simulink model "hybrid_pv_wind_islanding"  (R2024b)
settings: Solver=FixedStepDiscrete  StartTime=0.0  StopTime=1.0  FixedStep=P.Ts  RelTol=1e-3
model workspace (MAT data in the model file):
  P.Sn = 20000
  P.Vll = 400
  P.fg = 50
  P.wg = 314.159265359
  P.Vdc = 800
  P.fsw = 10000
  P.Ts = 2e-06
  P.In = 28.8675134595
  P.Ipk = 40.8248290464
  P.Vpk = 326.598632371
  P.logDecim = 10
  P.Zb = 8
  P.Lb = 0.0254647908947
  P.Cb = 0.00039788735773
  P.pv.Nser = 10
  P.pv.Npar = 5
  P.pv.Vmp = 290
  P.pv.Pstc = 10657.5
  P.pv.G0 = 1000
  P.pv.G1 = 1000
  P.pv.tStep = 1000000
  P.pv.T = 25
  P.pv.Tmppt = 0.01
  P.pv.dD = 0.003
  P.pv.D0 = 0.6375
  P.pv.Dmin = 0.45
  P.pv.Dmax = 0.8
  P.wind.R = 2.7072
  P.wind.rho = 1.225
  P.wind.CpMax = 0.411
  P.wind.lamOpt = 7.954
  P.wind.v0 = 12
  P.wind.v1 = 12
  P.wind.tStep = 1000000
  P.wind.Kopt = 0.228529744693
  P.wind.wm0 = 35.2570921986
  P.wind.Prated = 10015.7207747
  P.wind.J = 10
  P.wind.pp = 4
  P.wind.Ls = 0.003
  P.wind.Imax = 90
  P.wind.KpI = 0.04
  P.wind.KiI = 12
  P.wind.D0 = 0.76
  P.lcl.ripple = 0.2
  P.lcl.L1 = 0.0016
  P.lcl.L2 = 0.0008
  P.lcl.Cf = 1.5e-05
  P.lcl.wres = 11180.3398875
  P.lcl.fres = 1779.40635854
  P.lcl.Rd = 1.98761598
  P.lcl.R1 = 0.001
  P.lcl.R2 = 0.001
  P.grid.scr = 10
  P.grid.xr = 3
  P.grid.R = 0.252982212813
  P.grid.L = 0.00241580218102
  P.pll.wn = 188.495559215
  P.pll.zeta = 0.707
  P.pll.Kp = 0.816086456932
  P.pll.Ki = 108.789726356
  P.pll.Tf = 0.00795774715459
  P.ctrl.KpI = 6
  P.ctrl.KiI = 1000
  P.ctrl.KpV = 0.5
  P.ctrl.KiV = 10
  P.ctrl.Ilim = 61.2372435696
  P.prot.uv = 0.88
  P.prot.ov = 1.1
  P.prot.uf = 49.3
  P.prot.of = 50.5
  P.prot.rocof = 2
  P.prot.Trocof = 0.001
  P.prot.tBlank = 0.3
  P.load.Qf = 1
  P.load.P = 20000
  P.load.QL = 20000
  P.load.QC = 20000
  P.tIsland = 1000000
  P.check.Cf_pct_of_Cb = 3.76991118431
  P.check.Ltot_pu = 0.0942477796077
  P.check.fres_in_range = 1
  P.check.fres_with_grid = 1257.19940734
undefined symbols (not defined in the file): DiscIntNeverNeededParam
libraries: spsSeriesRLCBranchLib x14, spsIGBTDiodeLib x8, slpidlib x5, simulink x4, spsThreePhaseBreakerLib x2, spsDiodeLib x2, spsAlphaBetaZerotodq0Lib x2, eeGeneralControl x2, spsThreePhaseVIMeasurementLib x2, spsVoltageMeasurementLib x2, spsMeanLib x1, spsabctoAlphaBetaZeroLib x1
settings Model: LastModifiedBy=subas
settings SolverCC: AlgebraicLoopSolver=LineSearch
settings DataIOCC: ReturnWorkspaceOutputs=off
settings DebuggingCC: AlgebraicLoopMsg=none  ArithmeticOperatorsInVariantConditions=warning
settings ModelReferenceCC: EnableRefExpFcnMdlSchedulingChecks=on
settings SFSimCC: SimUseLocalCustomCode=off  CustomCodeUndefinedFunction=UseInterfaceOnly
settings RTWCC: RTWUseLocalCustomCode=off  GPUComputeCapability=3.5

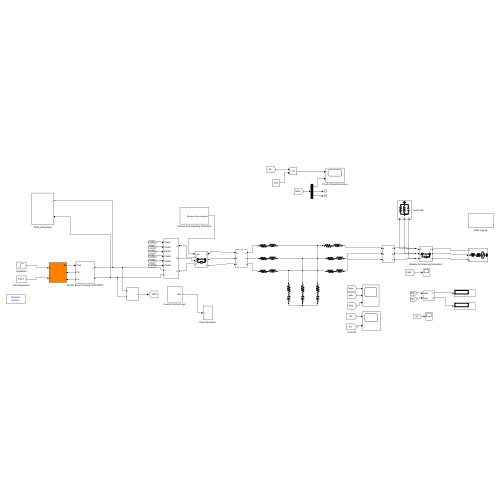
[thumbnail: Simulink's stored preview of the top-level diagram]
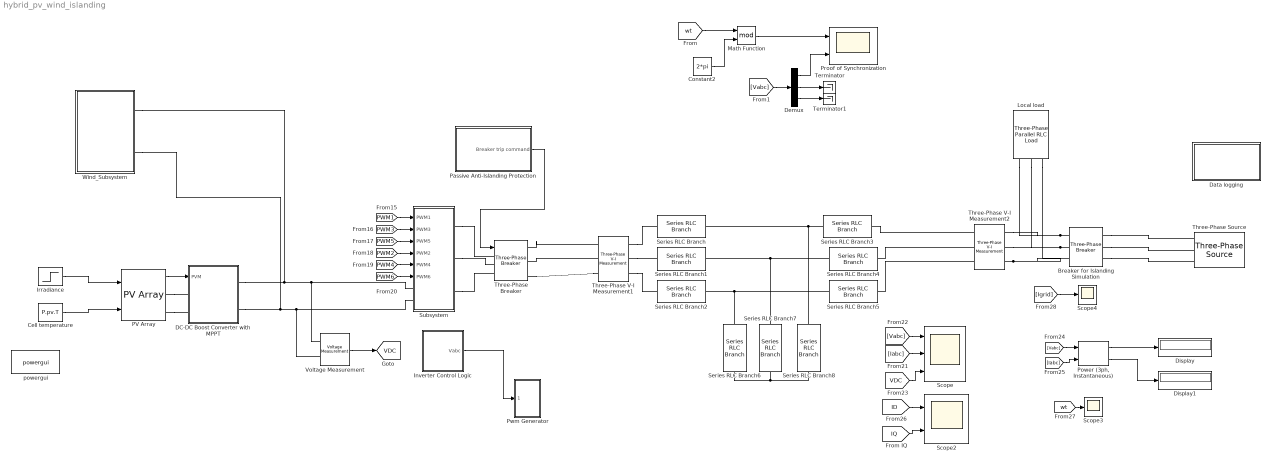
== system hybrid_pv_wind_islanding ==
  Breaker for Islanding Simulation : spsThreePhaseBreakerLib/Three-Phase Breaker  InitialState=closed  SwitchA=on  SwitchB=on  SwitchC=on  SwitchTimes=[P.tIsland]  External=off  BreakerResistance=0.01  SnubberResistance=1e6  SnubberCapacitance=inf  Measurements=None
  Cell temperature : Constant  Value=P.pv.T
  Constant2 : Constant  Value=2*pi
  DC-DC Boost Converter with MPPT : Subsystem
  Data logging : Subsystem
  Demux : Demux  Outputs=3
  Display : Display
  Display1 : Display
  Inverter Control Logic : Subsystem
  Irradiance : Step  Time=P.pv.tStep  Before=P.pv.G0  After=P.pv.G1  SampleTime=0
  Local load : spsThreePhaseParallelRLCLoadLib/Three-Phase Parallel RLC Load  LConnTagsString=A|B|C  Configuration=Y (grounded)  NominalVoltage=P.Vll  Vabc=[1e3 1e3 1e3]  Vabcp=[1e3 1e3 1e3]  NominalFrequency=P.fg  UnbalancedPower=off  ActivePower=P.load.P  InductivePower=P.load.QL  CapacitivePower=P.load.QC  Pabc=[10e3 9e3 11e3]  QLabc=[100 90 110]  QCabc=[100 90 110]  Pabcp=[10e3 9e3 11e3]  QLabcp=[100 90 110]  QCabcp=[100 90 110]  Measurements=None  LoadType=constant Z
  Math Function : Math  Operator=mod  SignedPower=on
  PV Array : spsPVArrayLib/PV Array  Npar=P.pv.Npar  Nser=P.pv.Nser  PlotType=array @ 1000 W/m2 & specified temperatures  S_vec="[ 1000  500  100 ]"  Temp_C_vec="[ 45 25  ]"  ModuleName=User-defined  PlotWhenSelected=off  Pm=213.15  Ncell=60  Voc=36.3  Isc=7.84  Vm=29  Im=7.35  beta_Voc_pc=-0.36099  alpha_Isc_pc=0.102  beta_Voc=-0.13104  alpha_Isc=0.0079968  IL=7.8654  I0=2.9273e-10  nI=0.98119  Rsh=313.0553  Rs=0.39381  RobustModel=off  RobustCellTemperature=313.3991  BAL=on  Tc=1e-6  Tfilter=5e-5
  Passive Anti-Islanding Protection : Subsystem
  "Power (3ph, Instantaneous)" : spsPower3phInstantaneousLib/Power (3ph, Instantaneous)
  Proof of Synchronization : Scope  NumInputPorts=2
  "Pwm Generator " : Subsystem
  Scope : Scope  NumInputPorts=3
  Scope2 : Scope  NumInputPorts=2
  Scope3 : Scope
  Scope4 : Scope
  Series RLC Branch : spsSeriesRLCBranchLib/Series RLC Branch  LConnTagsString=__new0  RConnTagsString=__new0  BranchType=RL  Resistance=P.lcl.R1  Inductance=P.lcl.L1  SetiL0=off  InitialCurrent=0  Capacitance=1e-6  Setx0=off  InitialVoltage=0  Measurements=None
  Series RLC Branch1 : spsSeriesRLCBranchLib/Series RLC Branch  LConnTagsString=__new0  RConnTagsString=__new0  BranchType=RL  Resistance=P.lcl.R1  Inductance=P.lcl.L1  SetiL0=off  InitialCurrent=0  Capacitance=1e-6  Setx0=off  InitialVoltage=0  Measurements=None
  Series RLC Branch2 : spsSeriesRLCBranchLib/Series RLC Branch  LConnTagsString=__new0  RConnTagsString=__new0  BranchType=RL  Resistance=P.lcl.R1  Inductance=P.lcl.L1  SetiL0=off  InitialCurrent=0  Capacitance=1e-6  Setx0=off  InitialVoltage=0  Measurements=None
  Series RLC Branch3 : spsSeriesRLCBranchLib/Series RLC Branch  LConnTagsString=__new0  RConnTagsString=__new0  BranchType=RL  Resistance=P.lcl.R2  Inductance=P.lcl.L2  SetiL0=off  InitialCurrent=10  Capacitance=1e-6  Setx0=off  InitialVoltage=0  Measurements=None
  Series RLC Branch4 : spsSeriesRLCBranchLib/Series RLC Branch  LConnTagsString=__new0  RConnTagsString=__new0  BranchType=RL  Resistance=P.lcl.R2  Inductance=P.lcl.L2  SetiL0=off  InitialCurrent=10  Capacitance=1e-6  Setx0=off  InitialVoltage=0  Measurements=None
  Series RLC Branch5 : spsSeriesRLCBranchLib/Series RLC Branch  LConnTagsString=__new0  RConnTagsString=__new0  BranchType=RL  Resistance=P.lcl.R2  Inductance=P.lcl.L2  SetiL0=off  InitialCurrent=10  Capacitance=1e-6  Setx0=off  InitialVoltage=0  Measurements=None
  Series RLC Branch6 : spsSeriesRLCBranchLib/Series RLC Branch  LConnTagsString=__new0  RConnTagsString=__new0  BranchType=RC  Resistance=P.lcl.Rd  Inductance=1000e-3  SetiL0=off  InitialCurrent=0  Capacitance=P.lcl.Cf  Setx0=off  InitialVoltage=0  Measurements=None
  Series RLC Branch7 : spsSeriesRLCBranchLib/Series RLC Branch  LConnTagsString=__new0  RConnTagsString=__new0  BranchType=RC  Resistance=P.lcl.Rd  Inductance=1000e-3  SetiL0=off  InitialCurrent=0  Capacitance=P.lcl.Cf  Setx0=off  InitialVoltage=0  Measurements=None
  Series RLC Branch8 : spsSeriesRLCBranchLib/Series RLC Branch  LConnTagsString=__new0  RConnTagsString=__new0  BranchType=RC  Resistance=P.lcl.Rd  Inductance=1000e-3  SetiL0=off  InitialCurrent=0  Capacitance=P.lcl.Cf  Setx0=off  InitialVoltage=0  Measurements=None
  Subsystem : Subsystem
  Terminator : Terminator
  Terminator1 : Terminator
  Three-Phase V-I Measurement1 : spsThreePhaseVIMeasurementLib/Three-Phase V-I Measurement  VoltageMeasurement=no  SetLabelV=off  LabelV=Vabc  Vpu=off  VpuLL=off  CurrentMeasurement=yes  SetLabelI=on  LabelI=Iabc  Ipu=off  Pbase=100e6  Vbase=500e3  OutputType=Complex  PhasorSimulation=off  PSBequivalent=0
  Three-Phase V-I Measurement2 : spsThreePhaseVIMeasurementLib/Three-Phase V-I Measurement  VoltageMeasurement=phase-to-ground  SetLabelV=on  LabelV=Vabc  Vpu=off  VpuLL=off  CurrentMeasurement=yes  SetLabelI=on  LabelI=Igrid  Ipu=off  Pbase=100e6  Vbase=500e3  OutputType=Complex  PhasorSimulation=off  PSBequivalent=0
  Three-Phase Breaker : spsThreePhaseBreakerLib/Three-Phase Breaker  InitialState=closed  SwitchA=on  SwitchB=on  SwitchC=on  SwitchTimes=[9999]  External=on  BreakerResistance=0.01  SnubberResistance=1e6  SnubberCapacitance=inf  Measurements=None
  Three-Phase Source : spsThreePhaseSourceLib/Three-Phase Source  InternalConnection=Yg  VoltagePhases=off  Voltage=P.Vll  PhaseAngle=0  Voltage_phases=[25e3 25e3 25e3]/sqrt(3)  PhaseAngles_phases=[0 -120 +120]  Frequency=P.fg  NonIdealSource=on  SpecifyImpedance=off  Resistance=P.grid.R  Inductance=P.grid.L  ShortCircuitLevel=10e-6  BaseVoltage=400  XRratio=7  BusType=swing  Pref=10e3  Qref=0  Prefabc=[10e3, 10e3, 10e3]  Qrefabc=[0, 0, 0]  Qmin=-inf  Qmax=inf
  Voltage Measurement : spsVoltageMeasurementLib/Voltage Measurement  PhasorSimulation=off  OutputType=Complex  PSBequivalent=0
  Wind_Subsystem : Subsystem
  powergui : spspowerguiLib/powergui  Priority=1  SimulationMode=Discrete  SampleTime=P.Ts  frequency=60  Iterations=50  frequencyindice=0  Pbase=100e6  ErrMax=1e-4  UnitsV=kV  UnitsW=MW  buscounter=0  FunctionMessages=off  echomessages=off  EnableUseOfTLC=off  CurrentSourceSwitches=off  DisableSnubberDevices=off  DisableRonSwitches=off  DisableVfSwitches=off  DisplayEquations=off  AutomaticDiscreteSolvers=off  SolverType=Tustin/Backward Euler (TBE)  Interpol=off  ExternalGateDelay=off  methode=off  Ts=100  x0status=blocks  SPID=off  SwTol=0  HookPort=off  NonlinearTolerance=1e-4  nMaxIteration=100  ContinueOnMaxIteration=off  RestoreLinks=warning  ResistiveCurrentMeasurement=off  Frange=[0:2:500]  Ylog=off  Xlog=on  ShowGrid=off  save=off  variable=ZData  structure=Grid_current  ZoomFFT=off  StartTime=0.4  cycles=5  DisplayStyle=1  fundamental=50  FreqAxis=off  MaxFrequency=1000  frequencyindicesteady=1  RmsSteady=1  display=off
  tag scope: VDC=global
  wires:
  Voltage Measurement/1 -> [VDC]
  [PWM6] -> Subsystem/6(PWM6)
  [PWM1] -> Subsystem/1(PWM1)
  "Power (3ph, Instantaneous)"/1 -> Display/1
  PV Array/1 -> DC-DC Boost Converter with MPPT/1("PVM ")
  [Iabc] -> "Power (3ph, Instantaneous)"/2
  [PWM3] -> Subsystem/2(PWM3)
  [Igrid] -> Scope4/1
  Inverter Control Logic/1(Vabc) -> "Pwm Generator "/1(1)
  [PWM4] -> Subsystem/5(PWM4)
  [Vabc] -> Scope/1
  [Vabc] -> "Power (3ph, Instantaneous)"/1
  [ID] -> Scope2/1
  "Power (3ph, Instantaneous)"/2 -> Display1/1
  [wt] -> Scope3/1
  [PWM2] -> Subsystem/4(PWM2)
  [VDC] -> Scope/3
  [PWM5] -> Subsystem/3(PWM5)
  [Iabc] -> Scope/2
  Passive Anti-Islanding Protection/1("Breaker trip command ") -> Three-Phase Breaker/1
  Demux/1 -> Proof of Synchronization/2
  Demux/2 -> Terminator/1
  Constant2/1 -> Math Function/2
  [wt] -> Math Function/1
  Math Function/1 -> Proof of Synchronization/1
  [Vabc] -> Demux/1
  Demux/3 -> Terminator1/1
  Irradiance/1 -> PV Array/1
  Cell temperature/1 -> PV Array/2
  [IQ] -> Scope2/2
  connections:
  Series RLC Branch7/RConn1 -- Series RLC Branch8/RConn1 -- Series RLC Branch6/RConn1
  Series RLC Branch8/LConn1 -- Series RLC Branch/RConn1 -- Series RLC Branch3/LConn1
  Series RLC Branch7/LConn1 -- Series RLC Branch1/RConn1 -- Series RLC Branch4/LConn1
  Series RLC Branch6/LConn1 -- Series RLC Branch2/RConn1 -- Series RLC Branch5/LConn1
  PV Array/RConn1 -- DC-DC Boost Converter with MPPT/LConn1
  Three-Phase V-I Measurement1/RConn3 -- Series RLC Branch2/LConn1
  Three-Phase V-I Measurement1/RConn1 -- Series RLC Branch/LConn1
  PV Array/RConn2 -- DC-DC Boost Converter with MPPT/LConn2
  Three-Phase V-I Measurement1/RConn2 -- Series RLC Branch1/LConn1
  DC-DC Boost Converter with MPPT/RConn1 -- Wind_Subsystem/RConn1 -- Subsystem/LConn1 -- Voltage Measurement/LConn1
  DC-DC Boost Converter with MPPT/RConn2 -- Wind_Subsystem/RConn2 -- Subsystem/LConn2 -- Voltage Measurement/LConn2
  Subsystem/RConn1 -- Three-Phase Breaker/LConn1
  Subsystem/RConn2 -- Three-Phase Breaker/LConn2
  Subsystem/RConn3 -- Three-Phase Breaker/LConn3
  Three-Phase Breaker/RConn1 -- Three-Phase V-I Measurement1/LConn1
  Three-Phase V-I Measurement1/LConn2 -- Three-Phase Breaker/RConn2
  Three-Phase Breaker/RConn3 -- Three-Phase V-I Measurement1/LConn3
  Breaker for Islanding Simulation/LConn1 -- Three-Phase V-I Measurement2/LConn1 -- Local load/LConn1
  Breaker for Islanding Simulation/LConn2 -- Three-Phase V-I Measurement2/LConn2 -- Local load/LConn2
  Three-Phase V-I Measurement2/LConn3 -- Breaker for Islanding Simulation/LConn3 -- Local load/LConn3
  Breaker for Islanding Simulation/RConn1 -- Three-Phase Source/RConn1
  Breaker for Islanding Simulation/RConn2 -- Three-Phase Source/RConn2
  Breaker for Islanding Simulation/RConn3 -- Three-Phase Source/RConn3
  Series RLC Branch3/RConn1 -- Three-Phase V-I Measurement2/RConn1
  Series RLC Branch4/RConn1 -- Three-Phase V-I Measurement2/RConn2
  Series RLC Branch5/RConn1 -- Three-Phase V-I Measurement2/RConn3

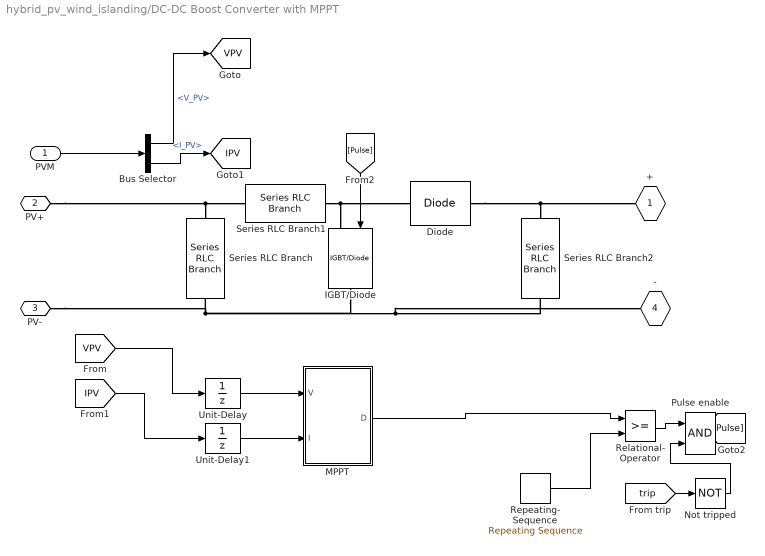
== system hybrid_pv_wind_islanding/DC-DC Boost Converter with MPPT ==
  "PVM " : Inport
  Bus Selector : BusSelector  OutputSignals=V_PV,I_PV
  Diode : spsDiodeLib/Diode  Ron=0.001  Lon=0  Vf=0.8  IC=0  UseSnubber=0  Rs=500  Cs=250e-9  Measurements=off
  IGBT/Diode : spsIGBTDiodeLib/IGBT//Diode  Ron=1e-3  Rs=1e5  Cs=inf  Measurements=off
  MPPT : MATLAB Function  TreatAsAtomicUnit=on
  Not tripped : Logic  Operator=NOT  AllPortsSameDT=off  OutDataTypeStr=boolean
  Pulse enable : Logic  AllPortsSameDT=off  OutDataTypeStr=boolean
  Relational- Operator : RelationalOperator  OutDataTypeStr=boolean  RndMeth=Simplest  InputSameDT=off
  Repeating- Sequence : simulink/Sources/Repeating Sequence  rep_seq_t=[0 0.0002]  rep_seq_y=[0 1]
  Series RLC Branch : spsSeriesRLCBranchLib/Series RLC Branch  LConnTagsString=__new0  RConnTagsString=__new0  BranchType=RC  Resistance=1e-3  Inductance=1e-3  SetiL0=off  InitialCurrent=0  Capacitance=1000e-6  Setx0=off  InitialVoltage=0  Measurements=None
  Series RLC Branch1 : spsSeriesRLCBranchLib/Series RLC Branch  LConnTagsString=__new0  RConnTagsString=__new0  BranchType=L  Resistance=1e-3  Inductance=1.5e-3  SetiL0=off  InitialCurrent=0  Capacitance=1000e-6  Setx0=off  InitialVoltage=0  Measurements=None
  Series RLC Branch2 : spsSeriesRLCBranchLib/Series RLC Branch  LConnTagsString=__new0  RConnTagsString=__new0  BranchType=C  Resistance=1e-3  Inductance=1e-3  SetiL0=off  InitialCurrent=0  Capacitance=3227e-6  Setx0=on  InitialVoltage=P.Vdc  Measurements=None
  Unit-Delay : UnitDelay  SampleTime=P.pv.Tmppt  HasFrameUpgradeWarning=on
  Unit-Delay1 : UnitDelay  SampleTime=P.pv.Tmppt  HasFrameUpgradeWarning=on
  + : PMIOPort  Side=Right
  PV+ : PMIOPort  Port=2  Side=Left
  PV- : PMIOPort  Port=3  Side=Left
  - : PMIOPort  Port=4  Side=Right
  tag scope: IPV=global, VPV=global
  wires:
  [Pulse] -> IGBT/Diode/1
  Bus Selector/1 -> [VPV]  "<V_PV>"
  Bus Selector/2 -> [IPV]  "<I_PV>"
  "PVM "/1 -> Bus Selector/1
  [VPV] -> Unit-Delay/1
  Unit-Delay/1 -> MPPT/1(V)
  Repeating- Sequence/1 -> Relational- Operator/2
  Unit-Delay1/1 -> MPPT/2(I)
  [IPV] -> Unit-Delay1/1
  MPPT/1(D) -> Relational- Operator/1
  [trip] -> Not tripped/1
  Relational- Operator/1 -> Pulse enable/1
  Not tripped/1 -> Pulse enable/2
  Pulse enable/1 -> [Pulse]
  connections:
  Diode/RConn1 -- +/RConn1 -- Series RLC Branch2/LConn1
  Series RLC Branch/RConn1 -- PV-/RConn1 -- -/RConn1 -- Series RLC Branch2/RConn1 -- IGBT/Diode/RConn1
  Series RLC Branch1/LConn1 -- Diode/LConn1 -- IGBT/Diode/LConn1
  Series RLC Branch/LConn1 -- PV+/RConn1 -- Series RLC Branch1/RConn1

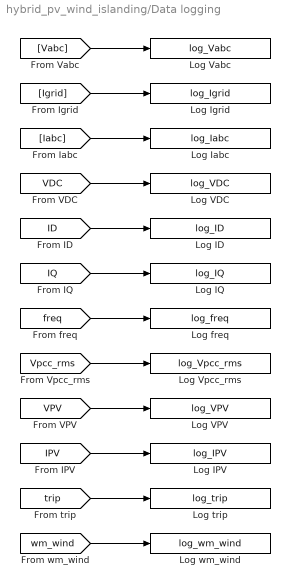
== system hybrid_pv_wind_islanding/Data logging ==
  Log ID : ToWorkspace  VariableName=log_ID  SaveFormat=Timeseries  SampleTime=-1
      settings: Decimation=P.logDecim
  Log IPV : ToWorkspace  VariableName=log_IPV  SaveFormat=Timeseries  SampleTime=-1
      settings: Decimation=P.logDecim
  Log IQ : ToWorkspace  VariableName=log_IQ  SaveFormat=Timeseries  SampleTime=-1
      settings: Decimation=P.logDecim
  Log Iabc : ToWorkspace  VariableName=log_Iabc  SaveFormat=Timeseries  SampleTime=-1
      settings: Decimation=P.logDecim
  Log Igrid : ToWorkspace  VariableName=log_Igrid  SaveFormat=Timeseries  SampleTime=-1
      settings: Decimation=P.logDecim
  Log VDC : ToWorkspace  VariableName=log_VDC  SaveFormat=Timeseries  SampleTime=-1
      settings: Decimation=P.logDecim
  Log VPV : ToWorkspace  VariableName=log_VPV  SaveFormat=Timeseries  SampleTime=-1
      settings: Decimation=P.logDecim
  Log Vabc : ToWorkspace  VariableName=log_Vabc  SaveFormat=Timeseries  SampleTime=-1
      settings: Decimation=P.logDecim
  Log Vpcc_rms : ToWorkspace  VariableName=log_Vpcc_rms  SaveFormat=Timeseries  SampleTime=-1
      settings: Decimation=P.logDecim
  Log freq : ToWorkspace  VariableName=log_freq  SaveFormat=Timeseries  SampleTime=-1
      settings: Decimation=P.logDecim
  Log trip : ToWorkspace  VariableName=log_trip  SaveFormat=Timeseries  SampleTime=-1
      settings: Decimation=P.logDecim
  Log wm_wind : ToWorkspace  VariableName=log_wm_wind  SaveFormat=Timeseries  SampleTime=-1
      settings: Decimation=P.logDecim
  wires:
  [Vabc] -> Log Vabc/1
  [Igrid] -> Log Igrid/1
  [Iabc] -> Log Iabc/1
  [VDC] -> Log VDC/1
  [ID] -> Log ID/1
  [IQ] -> Log IQ/1
  [freq] -> Log freq/1
  [Vpcc_rms] -> Log Vpcc_rms/1
  [VPV] -> Log VPV/1
  [IPV] -> Log IPV/1
  [trip] -> Log trip/1
  [wm_wind] -> Log wm_wind/1

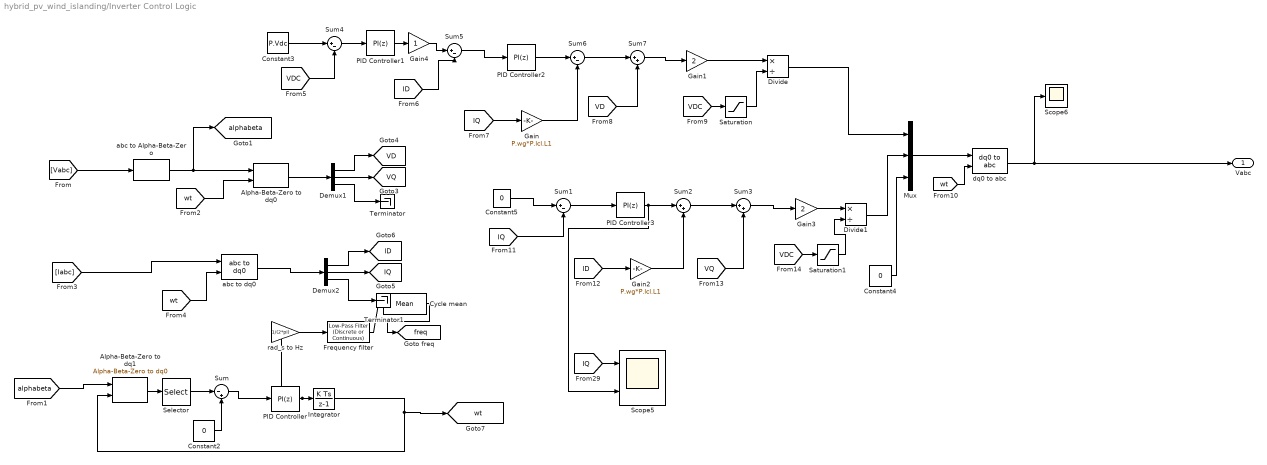
== system hybrid_pv_wind_islanding/Inverter Control Logic ==
  Alpha-Beta-Zero to dq0 : spsAlphaBetaZerotodq0Lib/Alpha-Beta-Zero to dq0  Alignment=90 degrees behind phase A axis
  Alpha-Beta-Zero to dq1 : spsAlphaBetaZerotodq0Lib/Alpha-Beta-Zero to dq0  Alignment=90 degrees behind phase A axis
  Constant2 : Constant  Value=0
  Constant3 : Constant  Value=P.Vdc
  Constant4 : Constant  Value=0
  Constant5 : Constant  Value=0
  Cycle mean : spsMeanLib/Mean  Freq=P.fg  Vinit=P.fg  Ts=P.Ts
  Demux1 : Demux  Outputs=3
  Demux2 : Demux  Outputs=3
  Divide : Product  Inputs=*/
  Divide1 : Product  Inputs=*/
  Frequency filter : eeGeneralControl/Low-Pass Filter (Discrete or Continuous)  K=1  T=P.pll.Tf  B=inf  A=-inf  init_option=Inherited from block input  x0=0  Ts=-1
  Gain : Gain  Gain=P.wg*P.lcl.L1
  Gain1 : Gain  Gain=2
  Gain2 : Gain  Gain=P.wg*P.lcl.L1
  Gain3 : Gain  Gain=2
  Gain4 : Gain
  Integrator : DiscreteIntegrator  SampleTime=-1  ICPrevOutput=DiscIntNeverNeededParam  ICPrevScaledInput=DiscIntNeverNeededParam
  Mux : Mux  Inputs=3
  PID Controller : slpidlib/PID Controller  Controller=PI  Form=Parallel  TimeDomain=Discrete-time  UseExternalTs=off  SampleTime=-1  IntegratorMethod=Forward Euler  FilterMethod=Forward Euler  ControllerParametersSource=internal  P=P.pll.Kp  I=P.pll.Ki  UseKiTs=off  D=0  UseExternalDerivativeSource=off  N=100  UseFilter=on  TunerSelectOption=Transfer Function Based (PID Tuner App)  InitialConditionSource=internal  InitialConditionForIntegrator=P.wg  InitialConditionForFilter=0  DifferentiatorICPrevScaledInput=0  ExternalReset=none  TrackingMode=off  Kt=1  LimitOutput=off  SatLimitsSource=internal  UpperSaturationLimit=inf  LowerSaturationLimit=-inf  LinearizeAsGain=on  AntiWindupMode=none  Kb=1  LimitIntegrator=off  UpperIntegratorSaturationLimit=inf  LowerIntegratorSaturationLimit=-inf  POutMin=[]  POutMax=[]  IOutMin=[]  IOutMax=[]  DOutMin=[]  DOutMax=[]  NOutMin=[]  NOutMax=[]  SumOutMin=[]  SumOutMax=[]  SaturationOutMin=[]  SaturationOutMax=[]  PParamMin=[]  PParamMax=[]  IParamMin=[]  IParamMax=[]  DParamMin=[]  DParamMax=[]  NParamMin=[]  NParamMax=[]  KbParamMin=[]  KbParamMax=[]  KtParamMin=[]  KtParamMax=[]  KbOutMin=[]  KbOutMax=[]  KtOutMin=[]  KtOutMax=[]  IntegratorOutMin=[]  IntegratorOutMax=[]  FilterOutMin=[]  FilterOutMax=[]  SumI1OutMin=[]  SumI1OutMax=[]  SumI2OutMin=[]  SumI2OutMax=[]  SumI3OutMin=[]  SumI3OutMax=[]  SumI4OutMin=[]  SumI4OutMax=[]  SumDOutMin=[]  SumDOutMax=[]  DifferentiatorOutMin=[]  DifferentiatorOutMax=[]  FilterDiffOutCoefMin=[]  FilterDiffOutCoefMax=[]  ReciprocalOutMin=[]  ReciprocalOutMax=[]  SumDenOutMin=[]  SumDenOutMax=[]  SumNumOutMin=[]  SumNumOutMax=[]  DivideOutMin=[]  DivideOutMax=[]  UdiffTsProdOutMin=[]  UdiffTsProdOutMax=[]  NTsProdOutMin=[]  NTsProdOutMax=[]  UintegralTsProdOutMin=[]  UintegralTsProdOutMax=[]  UngainTsProdOutMin=[]  UngainTsProdOutMax=[]  ClampingZeroOutDataTypeStr=Inherit: Inherit via back propagation  ClampingZeroOutMin=[]  ClampingZeroOutMax=[]  FilterDenConstantOutDataTypeStr=Inherit: Inherit via back propagation  FilterDenConstantOutMin=[]  FilterDenConstantOutMax=[]  PCopyOutDataTypeStr=Inherit: Inherit via back propagation  PCopyOutMin=[]  PCopyOutMax=[]  NCopyOutDataTypeStr=Inherit: Inherit via back propagation  NCopyOutMin=[]  NCopyOutMax=[]  IntegratorContinuousStateAttributes=''  IntegratorStateMustResolveToSignalObject=off  IntegratorRTWStateStorageClass=Auto  FilterContinuousStateAttributes=''  FilterStateMustResolveToSignalObject=off  FilterRTWStateStorageClass=Auto  ParallelPVariant=InternalParameters  IdealPVariant=Disabled  IVariant=InternalParameters  DVariant=Disabled  IntegratorVariant=Discrete  SatVariant=Disabled  AWVariant=Passthrough  PCopyVariant=Disabled  TRVariant=Disabled  FdbkBlocksVariant=Forward  IdealPFdbkVariant=Disabled  SatFdbkVariant=Disabled  DerivativeFilterVariant=Disabled  NVariant=Disabled  NCopyVariant=Disabled_SignalSpec  FilterICVariant=Disabled  IntegratorICVariant=InternalICs  ExternalResetVariant=Disabled  TRSumVariant=Passthrough  SumFdbkVariant=Disabled  SumVariant=Sum_PI  TsampFilterVariant=InternalTs  TsampNgainVariant=Passthrough  TsampIntegralVariant=Disabled_SignalSpec  ExternalSaturationOutDataTypeStr=Inherit: Same as second input  DerivativeSourceVariant=Disabled  PreIntVariant=InternalPreInt
  PID Controller1 : slpidlib/PID Controller  Controller=PI  Form=Parallel  TimeDomain=Discrete-time  UseExternalTs=off  SampleTime=-1  IntegratorMethod=Forward Euler  FilterMethod=Forward Euler  ControllerParametersSource=internal  P=P.ctrl.KpV  I=P.ctrl.KiV  UseKiTs=off  D=0  UseExternalDerivativeSource=off  N=100  UseFilter=on  TunerSelectOption=Transfer Function Based (PID Tuner App)  InitialConditionSource=internal  InitialConditionForIntegrator=0  InitialConditionForFilter=0  DifferentiatorICPrevScaledInput=0  ExternalReset=none  TrackingMode=off  Kt=1  LimitOutput=on  SatLimitsSource=internal  UpperSaturationLimit=P.ctrl.Ilim  LowerSaturationLimit=-P.ctrl.Ilim  LinearizeAsGain=on  AntiWindupMode=clamping  Kb=1  LimitIntegrator=off  UpperIntegratorSaturationLimit=inf  LowerIntegratorSaturationLimit=-inf  POutMin=[]  POutMax=[]  IOutMin=[]  IOutMax=[]  DOutMin=[]  DOutMax=[]  NOutMin=[]  NOutMax=[]  SumOutMin=[]  SumOutMax=[]  SaturationOutMin=[]  SaturationOutMax=[]  PParamMin=[]  PParamMax=[]  IParamMin=[]  IParamMax=[]  DParamMin=[]  DParamMax=[]  NParamMin=[]  NParamMax=[]  KbParamMin=[]  KbParamMax=[]  KtParamMin=[]  KtParamMax=[]  KbOutMin=[]  KbOutMax=[]  KtOutMin=[]  KtOutMax=[]  IntegratorOutMin=[]  IntegratorOutMax=[]  FilterOutMin=[]  FilterOutMax=[]  SumI1OutMin=[]  SumI1OutMax=[]  SumI2OutMin=[]  SumI2OutMax=[]  SumI3OutMin=[]  SumI3OutMax=[]  SumI4OutMin=[]  SumI4OutMax=[]  SumDOutMin=[]  SumDOutMax=[]  DifferentiatorOutMin=[]  DifferentiatorOutMax=[]  FilterDiffOutCoefMin=[]  FilterDiffOutCoefMax=[]  ReciprocalOutMin=[]  ReciprocalOutMax=[]  SumDenOutMin=[]  SumDenOutMax=[]  SumNumOutMin=[]  SumNumOutMax=[]  DivideOutMin=[]  DivideOutMax=[]  UdiffTsProdOutMin=[]  UdiffTsProdOutMax=[]  NTsProdOutMin=[]  NTsProdOutMax=[]  UintegralTsProdOutMin=[]  UintegralTsProdOutMax=[]  UngainTsProdOutMin=[]  UngainTsProdOutMax=[]  ClampingZeroOutDataTypeStr=Inherit: Inherit via back propagation  ClampingZeroOutMin=[]  ClampingZeroOutMax=[]  FilterDenConstantOutDataTypeStr=Inherit: Inherit via back propagation  FilterDenConstantOutMin=[]  FilterDenConstantOutMax=[]  PCopyOutDataTypeStr=Inherit: Inherit via back propagation  PCopyOutMin=[]  PCopyOutMax=[]  NCopyOutDataTypeStr=Inherit: Inherit via back propagation  NCopyOutMin=[]  NCopyOutMax=[]  IntegratorContinuousStateAttributes=''  IntegratorStateMustResolveToSignalObject=off  IntegratorRTWStateStorageClass=Auto  FilterContinuousStateAttributes=''  FilterStateMustResolveToSignalObject=off  FilterRTWStateStorageClass=Auto  ParallelPVariant=InternalParameters  IdealPVariant=Disabled  IVariant=InternalParameters  DVariant=Disabled  IntegratorVariant=Discrete  SatVariant=Enabled  AWVariant=DiscClampingParallel  PCopyVariant=Disabled  TRVariant=Disabled  FdbkBlocksVariant=Forward  IdealPFdbkVariant=Disabled  SatFdbkVariant=Disabled  DerivativeFilterVariant=Disabled  NVariant=Disabled  NCopyVariant=Disabled_SignalSpec  FilterICVariant=Disabled  IntegratorICVariant=InternalICs  ExternalResetVariant=Disabled  TRSumVariant=Passthrough  SumFdbkVariant=Disabled  SumVariant=Sum_PI  TsampFilterVariant=InternalTs  TsampNgainVariant=Passthrough  TsampIntegralVariant=Disabled_SignalSpec  ExternalSaturationOutDataTypeStr=Inherit: Same as second input  DerivativeSourceVariant=Disabled  PreIntVariant=InternalPreInt
  PID Controller2 : slpidlib/PID Controller  Controller=PI  Form=Parallel  TimeDomain=Discrete-time  UseExternalTs=off  SampleTime=-1  IntegratorMethod=Forward Euler  FilterMethod=Forward Euler  ControllerParametersSource=internal  P=P.ctrl.KpI  I=P.ctrl.KiI  UseKiTs=off  D=0  UseExternalDerivativeSource=off  N=100  UseFilter=on  TunerSelectOption=Transfer Function Based (PID Tuner App)  InitialConditionSource=internal  InitialConditionForIntegrator=0  InitialConditionForFilter=0  DifferentiatorICPrevScaledInput=0  ExternalReset=none  TrackingMode=off  Kt=1  LimitOutput=on  SatLimitsSource=internal  UpperSaturationLimit=400  LowerSaturationLimit=-400  LinearizeAsGain=on  AntiWindupMode=clamping  Kb=1  LimitIntegrator=off  UpperIntegratorSaturationLimit=inf  LowerIntegratorSaturationLimit=-inf  POutMin=[]  POutMax=[]  IOutMin=[]  IOutMax=[]  DOutMin=[]  DOutMax=[]  NOutMin=[]  NOutMax=[]  SumOutMin=[]  SumOutMax=[]  SaturationOutMin=[]  SaturationOutMax=[]  PParamMin=[]  PParamMax=[]  IParamMin=[]  IParamMax=[]  DParamMin=[]  DParamMax=[]  NParamMin=[]  NParamMax=[]  KbParamMin=[]  KbParamMax=[]  KtParamMin=[]  KtParamMax=[]  KbOutMin=[]  KbOutMax=[]  KtOutMin=[]  KtOutMax=[]  IntegratorOutMin=[]  IntegratorOutMax=[]  FilterOutMin=[]  FilterOutMax=[]  SumI1OutMin=[]  SumI1OutMax=[]  SumI2OutMin=[]  SumI2OutMax=[]  SumI3OutMin=[]  SumI3OutMax=[]  SumI4OutMin=[]  SumI4OutMax=[]  SumDOutMin=[]  SumDOutMax=[]  DifferentiatorOutMin=[]  DifferentiatorOutMax=[]  FilterDiffOutCoefMin=[]  FilterDiffOutCoefMax=[]  ReciprocalOutMin=[]  ReciprocalOutMax=[]  SumDenOutMin=[]  SumDenOutMax=[]  SumNumOutMin=[]  SumNumOutMax=[]  DivideOutMin=[]  DivideOutMax=[]  UdiffTsProdOutMin=[]  UdiffTsProdOutMax=[]  NTsProdOutMin=[]  NTsProdOutMax=[]  UintegralTsProdOutMin=[]  UintegralTsProdOutMax=[]  UngainTsProdOutMin=[]  UngainTsProdOutMax=[]  ClampingZeroOutDataTypeStr=Inherit: Inherit via back propagation  ClampingZeroOutMin=[]  ClampingZeroOutMax=[]  FilterDenConstantOutDataTypeStr=Inherit: Inherit via back propagation  FilterDenConstantOutMin=[]  FilterDenConstantOutMax=[]  PCopyOutDataTypeStr=Inherit: Inherit via back propagation  PCopyOutMin=[]  PCopyOutMax=[]  NCopyOutDataTypeStr=Inherit: Inherit via back propagation  NCopyOutMin=[]  NCopyOutMax=[]  IntegratorContinuousStateAttributes=''  IntegratorStateMustResolveToSignalObject=off  IntegratorRTWStateStorageClass=Auto  FilterContinuousStateAttributes=''  FilterStateMustResolveToSignalObject=off  FilterRTWStateStorageClass=Auto  ParallelPVariant=InternalParameters  IdealPVariant=Disabled  IVariant=InternalParameters  DVariant=Disabled  IntegratorVariant=Discrete  SatVariant=Enabled  AWVariant=DiscClampingParallel  PCopyVariant=Disabled  TRVariant=Disabled  FdbkBlocksVariant=Forward  IdealPFdbkVariant=Disabled  SatFdbkVariant=Disabled  DerivativeFilterVariant=Disabled  NVariant=Disabled  NCopyVariant=Disabled_SignalSpec  FilterICVariant=Disabled  IntegratorICVariant=InternalICs  ExternalResetVariant=Disabled  TRSumVariant=Passthrough  SumFdbkVariant=Disabled  SumVariant=Sum_PI  TsampFilterVariant=InternalTs  TsampNgainVariant=Passthrough  TsampIntegralVariant=Disabled_SignalSpec  ExternalSaturationOutDataTypeStr=Inherit: Same as second input  DerivativeSourceVariant=Disabled  PreIntVariant=InternalPreInt
  PID Controller3 : slpidlib/PID Controller  Controller=PI  Form=Parallel  TimeDomain=Discrete-time  UseExternalTs=off  SampleTime=-1  IntegratorMethod=Forward Euler  FilterMethod=Forward Euler  ControllerParametersSource=internal  P=P.ctrl.KpI  I=P.ctrl.KiI  UseKiTs=off  D=0  UseExternalDerivativeSource=off  N=100  UseFilter=on  TunerSelectOption=Transfer Function Based (PID Tuner App)  InitialConditionSource=internal  InitialConditionForIntegrator=0  InitialConditionForFilter=0  DifferentiatorICPrevScaledInput=0  ExternalReset=none  TrackingMode=off  Kt=1  LimitOutput=off  SatLimitsSource=internal  UpperSaturationLimit=inf  LowerSaturationLimit=-inf  LinearizeAsGain=on  AntiWindupMode=none  Kb=1  LimitIntegrator=off  UpperIntegratorSaturationLimit=inf  LowerIntegratorSaturationLimit=-inf  POutMin=[]  POutMax=[]  IOutMin=[]  IOutMax=[]  DOutMin=[]  DOutMax=[]  NOutMin=[]  NOutMax=[]  SumOutMin=[]  SumOutMax=[]  SaturationOutMin=[]  SaturationOutMax=[]  PParamMin=[]  PParamMax=[]  IParamMin=[]  IParamMax=[]  DParamMin=[]  DParamMax=[]  NParamMin=[]  NParamMax=[]  KbParamMin=[]  KbParamMax=[]  KtParamMin=[]  KtParamMax=[]  KbOutMin=[]  KbOutMax=[]  KtOutMin=[]  KtOutMax=[]  IntegratorOutMin=[]  IntegratorOutMax=[]  FilterOutMin=[]  FilterOutMax=[]  SumI1OutMin=[]  SumI1OutMax=[]  SumI2OutMin=[]  SumI2OutMax=[]  SumI3OutMin=[]  SumI3OutMax=[]  SumI4OutMin=[]  SumI4OutMax=[]  SumDOutMin=[]  SumDOutMax=[]  DifferentiatorOutMin=[]  DifferentiatorOutMax=[]  FilterDiffOutCoefMin=[]  FilterDiffOutCoefMax=[]  ReciprocalOutMin=[]  ReciprocalOutMax=[]  SumDenOutMin=[]  SumDenOutMax=[]  SumNumOutMin=[]  SumNumOutMax=[]  DivideOutMin=[]  DivideOutMax=[]  UdiffTsProdOutMin=[]  UdiffTsProdOutMax=[]  NTsProdOutMin=[]  NTsProdOutMax=[]  UintegralTsProdOutMin=[]  UintegralTsProdOutMax=[]  UngainTsProdOutMin=[]  UngainTsProdOutMax=[]  ClampingZeroOutDataTypeStr=Inherit: Inherit via back propagation  ClampingZeroOutMin=[]  ClampingZeroOutMax=[]  FilterDenConstantOutDataTypeStr=Inherit: Inherit via back propagation  FilterDenConstantOutMin=[]  FilterDenConstantOutMax=[]  PCopyOutDataTypeStr=Inherit: Inherit via back propagation  PCopyOutMin=[]  PCopyOutMax=[]  NCopyOutDataTypeStr=Inherit: Inherit via back propagation  NCopyOutMin=[]  NCopyOutMax=[]  IntegratorContinuousStateAttributes=''  IntegratorStateMustResolveToSignalObject=off  IntegratorRTWStateStorageClass=Auto  FilterContinuousStateAttributes=''  FilterStateMustResolveToSignalObject=off  FilterRTWStateStorageClass=Auto  ParallelPVariant=InternalParameters  IdealPVariant=Disabled  IVariant=InternalParameters  DVariant=Disabled  IntegratorVariant=Discrete  SatVariant=Disabled  AWVariant=Passthrough  PCopyVariant=Disabled  TRVariant=Disabled  FdbkBlocksVariant=Forward  IdealPFdbkVariant=Disabled  SatFdbkVariant=Disabled  DerivativeFilterVariant=Disabled  NVariant=Disabled  NCopyVariant=Disabled_SignalSpec  FilterICVariant=Disabled  IntegratorICVariant=InternalICs  ExternalResetVariant=Disabled  TRSumVariant=Passthrough  SumFdbkVariant=Disabled  SumVariant=Sum_PI  TsampFilterVariant=InternalTs  TsampNgainVariant=Passthrough  TsampIntegralVariant=Disabled_SignalSpec  ExternalSaturationOutDataTypeStr=Inherit: Same as second input  DerivativeSourceVariant=Disabled  PreIntVariant=InternalPreInt
  Saturation : Saturate  UpperLimit=1500  LowerLimit=50
  Saturation1 : Saturate  UpperLimit=1500  LowerLimit=50
  Scope5 : Scope  NumInputPorts=2
  Scope6 : Scope
  Selector : Selector  InputPortWidth=3  IndexOptions=Index vector (dialog)  Indices=2  OutputSizes=1
  Sum : Sum  Inputs=|-+
  Sum{1,4..6} (4 alike) : Sum  Inputs=|+-
  Sum2 : Sum  Inputs=|++
  Sum3 : Sum  Inputs=|++
  Sum7 : Sum  Inputs=|++
  Terminator : Terminator
  Terminator1 : Terminator
  abc to Alpha-Beta-Zero : spsabctoAlphaBetaZeroLib/abc to Alpha-Beta-Zero
  abc to dq0 : spsabctodq0Lib/abc to dq0  Alignment=90 degrees behind phase A axis
  dq0 to abc : spsdq0toabcLib/dq0 to abc  Alignment=90 degrees behind phase A axis
  rad_s to Hz : Gain  Gain=1/(2*pi)
  Vabc : Outport  VectorParamsAs1DForOutWhenUnconnected=off
  tag scope: ID=global, IQ=global, VD=global, VQ=global, alphabeta=global, freq=global, wt=global
  wires:
  Demux1/2 -> [VQ]
  Sum4/1 -> PID Controller1/1
  Constant3/1 -> Sum4/1
  Mux/1 -> dq0 to abc/1
  Sum5/1 -> PID Controller2/1
  Sum2/1 -> Sum3/1
  PID Controller3/1 -> Scope5/2, Sum2/1
  [alphabeta] -> Alpha-Beta-Zero to dq1/1
  [VDC] -> Saturation/1
  [ID] -> Gain2/1
  Gain1/1 -> Divide/1
  Demux2/3 -> Terminator1/1
  PID Controller2/1 -> Sum6/1
  PID Controller1/1 -> Gain4/1
  Divide1/1 -> Mux/2
  Gain4/1 -> Sum5/1
  Sum1/1 -> PID Controller3/1
  Selector/1 -> Sum/1
  Saturation1/1 -> Divide1/2
  [wt] -> dq0 to abc/2
  PID Controller/1 -> Integrator/1, rad_s to Hz/1
  Demux1/3 -> Terminator/1
  Integrator/1 -> [wt], Alpha-Beta-Zero to dq1/2
  Constant2/1 -> Sum/2
  Sum/1 -> PID Controller/1
  abc to Alpha-Beta-Zero/1 -> [alphabeta], Alpha-Beta-Zero to dq0/1
  Divide/1 -> Mux/1
  dq0 to abc/1 -> Vabc/1, Scope6/1
  Gain/1 -> Sum6/2
  Demux1/1 -> [VD]
  Alpha-Beta-Zero to dq0/1 -> Demux1/1
  [VQ] -> Sum3/2
  Sum6/1 -> Sum7/1
  [VDC] -> Saturation1/1
  Alpha-Beta-Zero to dq1/1 -> Selector/1
  Sum7/1 -> Gain1/1
  [VD] -> Sum7/2
  [IQ] -> Sum1/2
  abc to dq0/1 -> Demux2/1
  [IQ] -> Gain/1
  Constant5/1 -> Sum1/1
  Saturation/1 -> Divide/2
  Demux2/1 -> [ID]
  Sum3/1 -> Gain3/1
  [wt] -> Alpha-Beta-Zero to dq0/2
  [Iabc] -> abc to dq0/1
  [wt] -> abc to dq0/2
  Gain2/1 -> Sum2/2
  Gain3/1 -> Divide1/1
  Constant4/1 -> Mux/3
  Demux2/2 -> [IQ]
  [ID] -> Sum5/2
  [IQ] -> Scope5/1
  [Vabc] -> abc to Alpha-Beta-Zero/1
  [VDC] -> Sum4/2
  rad_s to Hz/1 -> Frequency filter/1
  Frequency filter/1 -> Cycle mean/1
  Cycle mean/1 -> [freq]

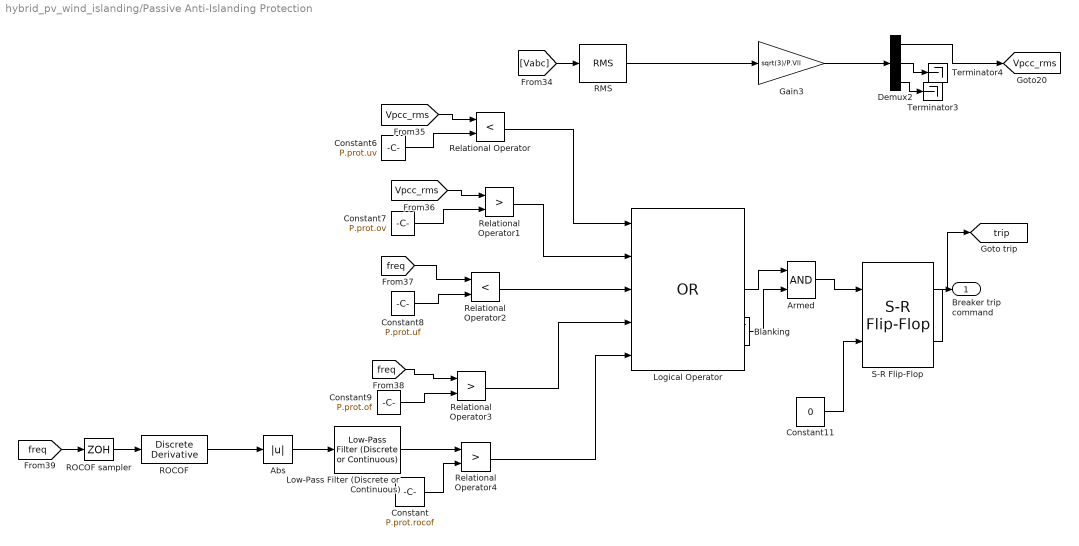
== system hybrid_pv_wind_islanding/Passive Anti-Islanding Protection ==
  Abs : Abs  SaturateOnIntegerOverflow=off
  Armed : Logic  AllPortsSameDT=off  OutDataTypeStr=boolean
  Blanking : Step  Time=P.prot.tBlank  SampleTime=P.Ts
  Constant : Constant  Value=P.prot.rocof
  Constant11 : Constant  Value=0  VectorParams1D=off  OutDataTypeStr=boolean
  Constant6 : Constant  Value=P.prot.uv
  Constant7 : Constant  Value=P.prot.ov
  Constant8 : Constant  Value=P.prot.uf
  Constant9 : Constant  Value=P.prot.of
  Demux2 : Demux  Outputs=3
  Gain3 : Gain  Gain=sqrt(3)/P.Vll
  Logical Operator : Logic  Operator=OR  Inputs=5  AllPortsSameDT=off  OutDataTypeStr=boolean
  Low-Pass Filter (Discrete or Continuous) : eeGeneralControl/Low-Pass Filter (Discrete or Continuous)  K=1  T=1/(2*pi*10)  B=inf  A=-inf  init_option=Inherited from block input  x0=0  Ts=-1
  RMS : spsRMSLib/RMS  TrueRMS=on  Freq=P.fg  RMSInit=120  Ts=P.Ts
  ROCOF : simulink/Discrete/Discrete Derivative  gainval=1.0  ICPrevScaledInput=0.0  OutMin=[]  OutMax=[]  OutDataType=fixdt(1, 16)  OutScaling=2^-10  DoSatur=off
  ROCOF sampler : ZeroOrderHold  SampleTime=P.prot.Trocof
  Relational Operator : RelationalOperator  Operator=<  OutDataTypeStr=boolean  RndMeth=Simplest  InputSameDT=off
  Relational Operator1 : RelationalOperator  Operator=>  OutDataTypeStr=boolean  RndMeth=Simplest  InputSameDT=off
  Relational Operator2 : RelationalOperator  Operator=<  OutDataTypeStr=boolean  RndMeth=Simplest  InputSameDT=off
  Relational Operator3 : RelationalOperator  Operator=>  OutDataTypeStr=boolean  RndMeth=Simplest  InputSameDT=off
  Relational Operator4 : RelationalOperator  Operator=>  OutDataTypeStr=boolean  RndMeth=Simplest  InputSameDT=off
  S-R Flip-Flop : simulink_extras/Flip Flops/S-R Flip-Flop  initial_condition=0
  Terminator3 : Terminator
  Terminator4 : Terminator
  "Breaker trip command " : Outport  VectorParamsAs1DForOutWhenUnconnected=off
  tag scope: Vpcc_rms=global, trip=global
  wires:
  RMS/1 -> Gain3/1
  Constant6/1 -> Relational Operator/2
  Constant7/1 -> Relational Operator1/2
  Abs/1 -> Low-Pass Filter (Discrete or Continuous)/1
  [Vpcc_rms] -> Relational Operator1/1
  Gain3/1 -> Demux2/1
  [Vabc] -> RMS/1
  [freq] -> Relational Operator3/1
  Low-Pass Filter (Discrete or Continuous)/1 -> Relational Operator4/1
  Constant11/1 -> S-R Flip-Flop/2
  Demux2/1 -> [Vpcc_rms]
  Constant8/1 -> Relational Operator2/2
  Constant/1 -> Relational Operator4/2
  Constant9/1 -> Relational Operator3/2
  [Vpcc_rms] -> Relational Operator/1
  Demux2/2 -> Terminator4/1
  Relational Operator1/1 -> Logical Operator/2
  Demux2/3 -> Terminator3/1
  Relational Operator3/1 -> Logical Operator/4
  Relational Operator/1 -> Logical Operator/1
  Relational Operator2/1 -> Logical Operator/3
  [freq] -> Relational Operator2/1
  Relational Operator4/1 -> Logical Operator/5
  [freq] -> ROCOF sampler/1
  ROCOF sampler/1 -> ROCOF/1
  ROCOF/1 -> Abs/1
  Logical Operator/1 -> Armed/1
  Blanking/1 -> Armed/2
  Armed/1 -> S-R Flip-Flop/1
  S-R Flip-Flop/2 -> "Breaker trip command "/1
  S-R Flip-Flop/1 -> [trip]

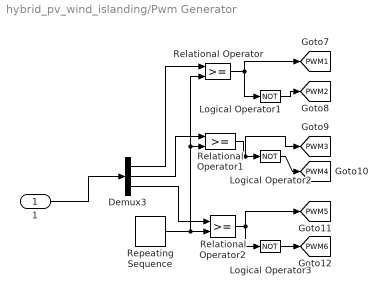
== system hybrid_pv_wind_islanding/Pwm Generator  ==
  1 : Inport
  Demux3 : Demux  Outputs=3
  Logical Operator1 : Logic  Operator=NOT  AllPortsSameDT=off  OutDataTypeStr=boolean
  Logical Operator2 : Logic  Operator=NOT  AllPortsSameDT=off  OutDataTypeStr=boolean
  Logical Operator3 : Logic  Operator=NOT  AllPortsSameDT=off  OutDataTypeStr=boolean
  Relational Operator : RelationalOperator  OutDataTypeStr=boolean  RndMeth=Simplest  InputSameDT=off
  Relational Operator1 : RelationalOperator  OutDataTypeStr=boolean  RndMeth=Simplest  InputSameDT=off
  Relational Operator2 : RelationalOperator  OutDataTypeStr=boolean  RndMeth=Simplest  InputSameDT=off
  Repeating Sequence : simulink/Sources/Repeating Sequence  rep_seq_t=[0 0.00005 0.0001]  rep_seq_y=[-1 1 -1]
  tag scope: PWM1=global, PWM2=global, PWM3=global, PWM4=global, PWM5=global, PWM6=global
  wires:
  Relational Operator/1 -> Logical Operator1/1, [PWM1]
  Demux3/2 -> Relational Operator1/1
  Demux3/1 -> Relational Operator/1
  Relational Operator1/1 -> [PWM3], Logical Operator2/1
  Repeating Sequence/1 -> Relational Operator1/2, Relational Operator/2, Relational Operator2/2
  Demux3/3 -> Relational Operator2/1
  1/1 -> Demux3/1
  Relational Operator2/1 -> [PWM5], Logical Operator3/1
  Logical Operator1/1 -> [PWM2]
  Logical Operator2/1 -> [PWM4]
  Logical Operator3/1 -> [PWM6]

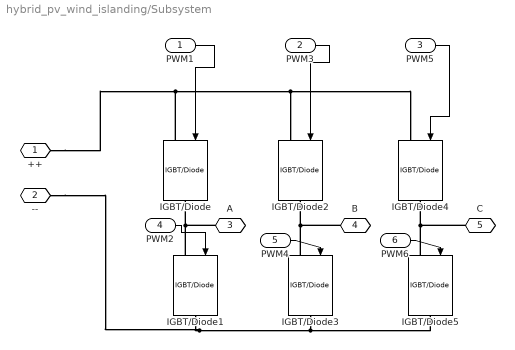
== system hybrid_pv_wind_islanding/Subsystem ==
  PWM1 : Inport
  PWM3 : Inport  Port=2
  PWM5 : Inport  Port=3
  PWM2 : Inport  Port=4
  PWM4 : Inport  Port=5
  PWM6 : Inport  Port=6
  IGBT/Diode{,1..5} (6 alike) : spsIGBTDiodeLib/IGBT//Diode  Ron=1e-3  Rs=1e5  Cs=inf  Measurements=off
  ++ : PMIOPort  Side=Left
  -- : PMIOPort  Port=2  Side=Left
  A : PMIOPort  Port=3  Side=Right
  B : PMIOPort  Port=4  Side=Right
  C : PMIOPort  Port=5  Side=Right
  wires:
  PWM1/1 -> IGBT/Diode/1
  PWM4/1 -> IGBT/Diode3/1
  PWM6/1 -> IGBT/Diode5/1
  PWM3/1 -> IGBT/Diode2/1
  PWM5/1 -> IGBT/Diode4/1
  PWM2/1 -> IGBT/Diode1/1
  connections:
  IGBT/Diode1/RConn1 -- --/RConn1 -- IGBT/Diode3/RConn1 -- IGBT/Diode5/RConn1
  IGBT/Diode3/LConn1 -- B/RConn1 -- IGBT/Diode2/RConn1
  IGBT/Diode1/LConn1 -- A/RConn1 -- IGBT/Diode/RConn1
  IGBT/Diode5/LConn1 -- C/RConn1 -- IGBT/Diode4/RConn1
  IGBT/Diode/LConn1 -- ++/RConn1 -- IGBT/Diode2/LConn1 -- IGBT/Diode4/LConn1

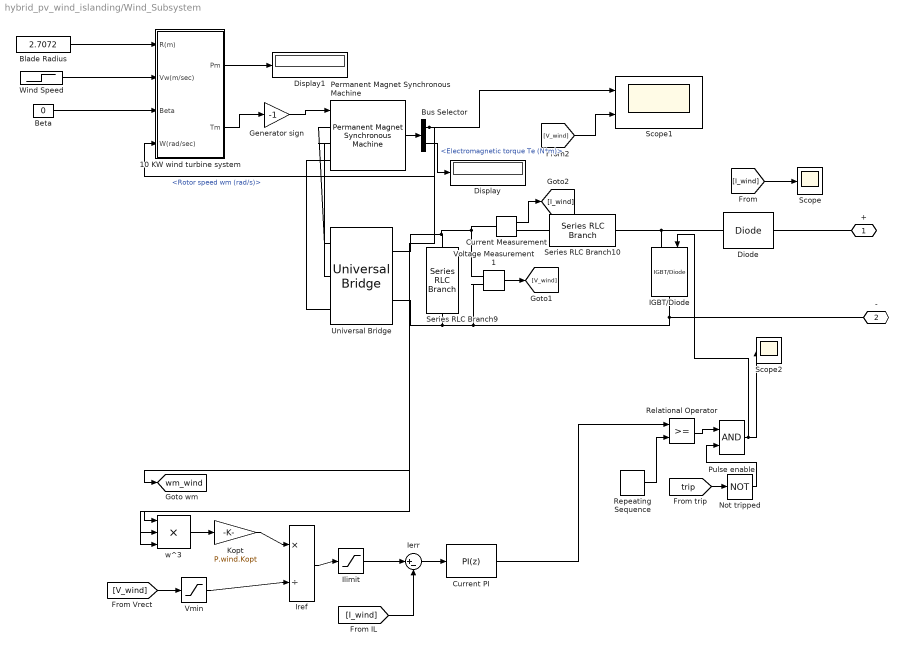
== system hybrid_pv_wind_islanding/Wind_Subsystem ==
  10 KW wind turbine system : Subsystem
  Beta : Constant  Value=0
  Blade Radius : Constant  Value=2.7072
  Bus Selector : BusSelector  OutputSignals=Rotor speed wm (rad/s),Electromagnetic torque Te (N*m)
  Current Measurement : spsCurrentMeasurementLib/Current Measurement  PhasorSimulation=off  OutputType=Complex  PSBequivalent=0
  Current PI : slpidlib/PID Controller  Controller=PI  Form=Parallel  TimeDomain=Discrete-time  UseExternalTs=off  SampleTime=-1  IntegratorMethod=Forward Euler  FilterMethod=Forward Euler  ControllerParametersSource=internal  P=P.wind.KpI  I=P.wind.KiI  UseKiTs=off  D=0  UseExternalDerivativeSource=off  N=100  UseFilter=on  TunerSelectOption=Transfer Function Based (PID Tuner App)  InitialConditionSource=internal  InitialConditionForIntegrator=P.wind.D0  InitialConditionForFilter=0  DifferentiatorICPrevScaledInput=0  ExternalReset=none  TrackingMode=off  Kt=1  LimitOutput=on  SatLimitsSource=internal  UpperSaturationLimit=0.92  LowerSaturationLimit=0  LinearizeAsGain=off  AntiWindupMode=clamping  Kb=1  LimitIntegrator=off  UpperIntegratorSaturationLimit=inf  LowerIntegratorSaturationLimit=-inf  POutMin=[]  POutMax=[]  IOutMin=[]  IOutMax=[]  DOutMin=[]  DOutMax=[]  NOutMin=[]  NOutMax=[]  SumOutMin=[]  SumOutMax=[]  SaturationOutMin=[]  SaturationOutMax=[]  PParamMin=[]  PParamMax=[]  IParamMin=[]  IParamMax=[]  DParamMin=[]  DParamMax=[]  NParamMin=[]  NParamMax=[]  KbParamMin=[]  KbParamMax=[]  KtParamMin=[]  KtParamMax=[]  KbOutMin=[]  KbOutMax=[]  KtOutMin=[]  KtOutMax=[]  IntegratorOutMin=[]  IntegratorOutMax=[]  FilterOutMin=[]  FilterOutMax=[]  SumI1OutMin=[]  SumI1OutMax=[]  SumI2OutMin=[]  SumI2OutMax=[]  SumI3OutMin=[]  SumI3OutMax=[]  SumI4OutMin=[]  SumI4OutMax=[]  SumDOutMin=[]  SumDOutMax=[]  DifferentiatorOutMin=[]  DifferentiatorOutMax=[]  FilterDiffOutCoefMin=[]  FilterDiffOutCoefMax=[]  ReciprocalOutMin=[]  ReciprocalOutMax=[]  SumDenOutMin=[]  SumDenOutMax=[]  SumNumOutMin=[]  SumNumOutMax=[]  DivideOutMin=[]  DivideOutMax=[]  UdiffTsProdOutMin=[]  UdiffTsProdOutMax=[]  NTsProdOutMin=[]  NTsProdOutMax=[]  UintegralTsProdOutMin=[]  UintegralTsProdOutMax=[]  UngainTsProdOutMin=[]  UngainTsProdOutMax=[]  ClampingZeroOutDataTypeStr=Inherit: Inherit via back propagation  ClampingZeroOutMin=[]  ClampingZeroOutMax=[]  FilterDenConstantOutDataTypeStr=Inherit: Inherit via back propagation  FilterDenConstantOutMin=[]  FilterDenConstantOutMax=[]  PCopyOutDataTypeStr=Inherit: Inherit via back propagation  PCopyOutMin=[]  PCopyOutMax=[]  NCopyOutDataTypeStr=Inherit: Inherit via back propagation  NCopyOutMin=[]  NCopyOutMax=[]  IntegratorContinuousStateAttributes=''  IntegratorStateMustResolveToSignalObject=off  IntegratorRTWStateStorageClass=Auto  FilterContinuousStateAttributes=''  FilterStateMustResolveToSignalObject=off  FilterRTWStateStorageClass=Auto  ParallelPVariant=InternalParameters  IdealPVariant=Disabled  IVariant=InternalParameters  DVariant=Disabled  IntegratorVariant=Discrete  SatVariant=Enabled  AWVariant=DiscClampingParallel  PCopyVariant=Disabled  TRVariant=Disabled  FdbkBlocksVariant=Forward  IdealPFdbkVariant=Disabled  SatFdbkVariant=Disabled  DerivativeFilterVariant=Disabled  NVariant=Disabled  NCopyVariant=Disabled_SignalSpec  FilterICVariant=Disabled  IntegratorICVariant=InternalICs  ExternalResetVariant=Disabled  TRSumVariant=Passthrough  SumFdbkVariant=Disabled  SumVariant=Sum_PI  TsampFilterVariant=InternalTs  TsampNgainVariant=Passthrough  TsampIntegralVariant=Disabled_SignalSpec  ExternalSaturationOutDataTypeStr=Inherit: Same as second input  DerivativeSourceVariant=Disabled  PreIntVariant=InternalPreInt
      settings: LibrarySourceBlock=simulink/Discrete/Discrete PID Controller
  Diode : spsDiodeLib/Diode  Ron=0.001  Lon=0  Vf=0.8  IC=0  UseSnubber=0  Rs=500  Cs=250e-9  Measurements=off
  Display : Display
  Display1 : Display
  Generator sign : Gain  Gain=-1
  IGBT/Diode : spsIGBTDiodeLib/IGBT//Diode  Ron=0.001  Rs=100  Cs=1e-6  Measurements=off
  Ierr : Sum  Inputs=|+-
  Ilimit : Saturate  UpperLimit=P.wind.Imax  LowerLimit=0
  Iref : Product  Inputs=*/
  Kopt : Gain  Gain=P.wind.Kopt
  Not tripped : Logic  Operator=NOT  AllPortsSameDT=off  OutDataTypeStr=boolean
  Permanent Magnet Synchronous Machine : spsPermanentMagnetSynchronousMachineLib/Permanent Magnet Synchronous Machine  NbPhases=3  FluxDistribution=Sinusoidal  RotorType=Round  MechanicalLoad=Torque Tm  PresetModel=No  ShowDetailedParameters=on  MeasurementBus=off  Resistance=0.05486  Inductance=P.wind.Ls  dqInductances=[P.wind.Ls P.wind.Ls]  La=0.000835  MachineConstant=Flux linkage established by magnets (V.s)  Flux=0.9  VoltageCst=652.9678  TorqueCst=5.4  Flat=120  Mechanical=[P.wind.J 0.008 P.wind.pp 0]  PolePairs=P.wind.pp  InitialConditions=[P.wind.wm0 0 0 0]  InitialConditions5ph=[0 0 0 0 0 0]  RefAngle=90 degrees behind phase A axis (modified Park)  IterativeDiscreteModel=Trapezoidal non iterative  TsBlock=-1  TsPowergui=0
  Pulse enable : Logic  AllPortsSameDT=off  OutDataTypeStr=boolean
  Relational Operator : RelationalOperator  OutDataTypeStr=boolean  RndMeth=Simplest  InputSameDT=off
  Repeating Sequence : simulink/Sources/Repeating Sequence  rep_seq_t="[0  0.0001]"  rep_seq_y=[0 1]
  Scope : Scope
  Scope1 : Scope  NumInputPorts=2
  Scope2 : Scope
  Series RLC Branch10 : spsSeriesRLCBranchLib/Series RLC Branch  LConnTagsString=__new0  RConnTagsString=__new0  BranchType=L  Resistance=2.3e-3  Inductance=10e-3  SetiL0=off  InitialCurrent=0  Capacitance=1e-6  Setx0=off  InitialVoltage=0  Measurements=None
  Series RLC Branch9 : spsSeriesRLCBranchLib/Series RLC Branch  LConnTagsString=__new0  RConnTagsString=__new0  BranchType=C  Resistance=1  Inductance=1e-3  SetiL0=off  InitialCurrent=0  Capacitance=2200e-6  Setx0=off  InitialVoltage=0  Measurements=None
  Universal Bridge : spsUniversalBridgeLib/Universal Bridge  Arms=3  SnubberResistance=5000  SnubberCapacitance=inf  Device=Diodes  Ron=0.001  Lon=0  ForwardVoltages="[  0  0  ]"  ForwardVoltage=0  GTOparameters=[ 10e-6 , 20e-6 ]  IGBTparameters=[ 1e-6 , 2e-6 ]  Measurements=None  Measurements_2=None  converterType=Rectifier
  Vmin : Saturate  UpperLimit=inf  LowerLimit=50
  Voltage Measurement1 : spsVoltageMeasurementLib/Voltage Measurement  PhasorSimulation=off  OutputType=Complex  PSBequivalent=0
  Wind Speed : Step  Time=P.wind.tStep  Before=P.wind.v0  After=P.wind.v1  SampleTime=0
  w^3 : Product  Inputs=3
  + : PMIOPort  Side=Right
  - : PMIOPort  Port=2  Side=Right
  tag scope: wm_wind=global
  wires:
  Bus Selector/1 -> Scope1/1, 10 KW wind turbine system/4(W(rad/sec)), w^3/1, w^3/2, w^3/3, [wm_wind]  "<Rotor speed wm (rad/s)>"
  [V_wind] -> Scope1/2
  Repeating Sequence/1 -> Relational Operator/2
  Permanent Magnet Synchronous Machine/1 -> Bus Selector/1
  Bus Selector/2 -> Display/1  "<Electromagnetic torque Te (N*m)>"
  Voltage Measurement1/1 -> [V_wind]
  Current Measurement/1 -> [I_wind]
  Beta/1 -> 10 KW wind turbine system/3(Beta)
  Blade Radius/1 -> 10 KW wind turbine system/1(R(m))
  10 KW wind turbine system/1(Pm) -> Display1/1
  Wind Speed/1 -> 10 KW wind turbine system/2(Vw(m/sec))
  [I_wind] -> Scope/1
  10 KW wind turbine system/2(Tm) -> Generator sign/1
  Generator sign/1 -> Permanent Magnet Synchronous Machine/1
  w^3/1 -> Kopt/1
  Kopt/1 -> Iref/1
  [V_wind] -> Vmin/1
  Vmin/1 -> Iref/2
  Iref/1 -> Ilimit/1
  Ilimit/1 -> Ierr/1
  [I_wind] -> Ierr/2
  Ierr/1 -> Current PI/1
  Current PI/1 -> Relational Operator/1
  [trip] -> Not tripped/1
  Relational Operator/1 -> Pulse enable/1
  Not tripped/1 -> Pulse enable/2
  Pulse enable/1 -> Scope2/1, IGBT/Diode/1
  connections:
  Series RLC Branch9/LConn1 -- Universal Bridge/RConn1 -- Voltage Measurement1/LConn1 -- Current Measurement/LConn1
  IGBT/Diode/RConn1 -- Voltage Measurement1/LConn2 -- Universal Bridge/RConn2 -- Series RLC Branch9/RConn1 -- -/RConn1
  Series RLC Branch10/RConn1 -- Diode/LConn1 -- IGBT/Diode/LConn1
  Diode/RConn1 -- +/RConn1
  Permanent Magnet Synchronous Machine/LConn2 -- Universal Bridge/LConn2
  Permanent Magnet Synchronous Machine/LConn1 -- Universal Bridge/LConn1
  Current Measurement/RConn1 -- Series RLC Branch10/LConn1
  Permanent Magnet Synchronous Machine/LConn3 -- Universal Bridge/LConn3

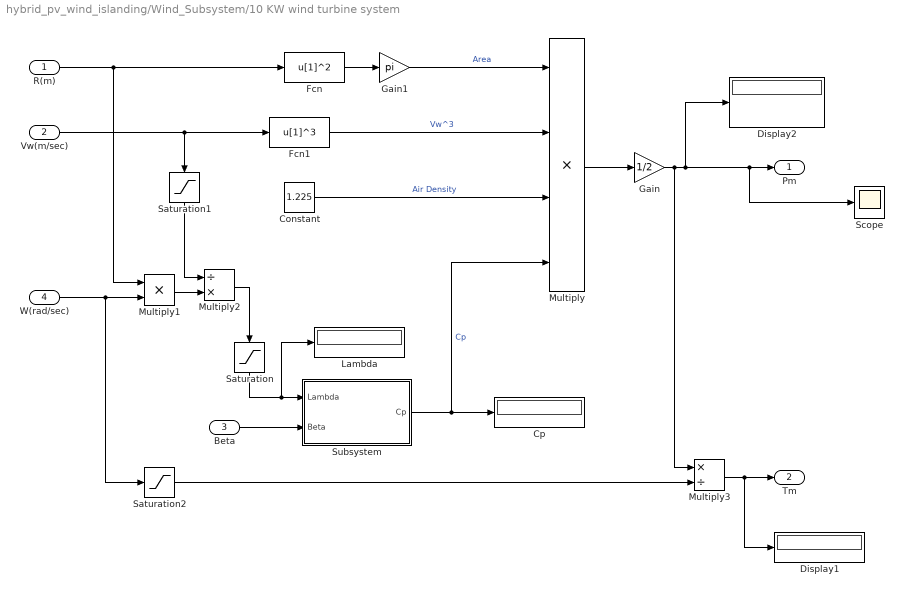
== system hybrid_pv_wind_islanding/Wind_Subsystem/10 KW wind turbine system ==
  R(m) : Inport
  Vw(m/sec) : Inport  Port=2
  Beta : Inport  Port=3
  W(rad/sec) : Inport  Port=4
  Constant : Constant  Value=1.225
  Cp : Display
  Display1 : Display
  Display2 : Display
  Fcn : Fcn  Expr=u[1]^2
  Fcn1 : Fcn  Expr=u[1]^3
  Gain : Gain  Gain=1/2
  Gain1 : Gain  Gain=pi
  Lambda : Display
  Multiply : Product  Inputs=4
  Multiply1 : Product
  Multiply2 : Product  Inputs=/*
  Multiply3 : Product  Inputs=*/
  Saturation : Saturate  UpperLimit=inf  LowerLimit=1e-6
  Saturation1 : Saturate  UpperLimit=inf  LowerLimit=1e-6
  Saturation2 : Saturate  UpperLimit=inf  LowerLimit=1e-6
  Scope : Scope
  Subsystem : Subsystem
  Pm : Outport  VectorParamsAs1DForOutWhenUnconnected=off
  Tm : Outport  Port=2  VectorParamsAs1DForOutWhenUnconnected=off
  wires:
  Gain/1 -> Multiply3/1, Display2/1, Scope/1, Pm/1
  Multiply/1 -> Gain/1
  Gain1/1 -> Multiply/1  "Area"
  Fcn1/1 -> Multiply/2  "Vw^3"
  Constant/1 -> Multiply/3  "Air Density"
  Subsystem/1(Cp) -> Cp/1, Multiply/4  "Cp"
  Fcn/1 -> Gain1/1
  R(m)/1 -> Multiply1/1, Fcn/1
  Vw(m/sec)/1 -> Fcn1/1, Saturation1/1
  Beta/1 -> Subsystem/2(Beta)
  W(rad/sec)/1 -> Saturation2/1, Multiply1/2
  Multiply1/1 -> Multiply2/2
  Multiply2/1 -> Saturation/1
  Saturation1/1 -> Multiply2/1
  Saturation2/1 -> Multiply3/2
  Multiply3/1 -> Display1/1, Tm/1
  Saturation/1 -> Lambda/1, Subsystem/1(Lambda)

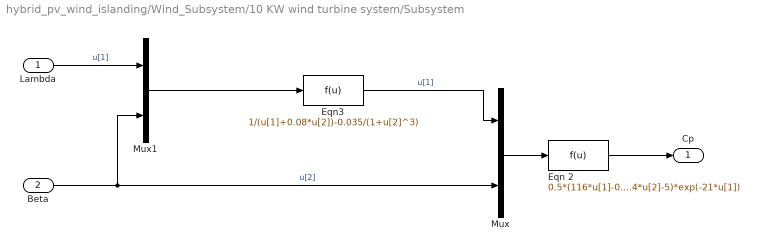
== system hybrid_pv_wind_islanding/Wind_Subsystem/10 KW wind turbine system/Subsystem ==
  Lambda : Inport
  Beta : Inport  Port=2
  Eqn 2 : Fcn  Expr=0.5*(116*u[1]-0.4*u[2]-5)*exp(-21*u[1])
  Eqn3 : Fcn  Expr=1/(u[1]+0.08*u[2])-0.035/(1+u[2]^3)
  Mux : Mux  Inputs=2
  Mux1 : Mux  Inputs=2
  Cp : Outport  VectorParamsAs1DForOutWhenUnconnected=off
  wires:
  Eqn 2/1 -> Cp/1
  Mux/1 -> Eqn 2/1
  Lambda/1 -> Mux1/1  "u[1]"
  Eqn3/1 -> Mux/1  "u[1]"
  Beta/1 -> Mux1/2, Mux/2  "u[2]"
  Mux1/1 -> Eqn3/1

== matlab function hybrid_pv_wind_islanding/DC-DC Boost Converter with MPPT/MPPT ==
  data: V input; D output; I input
function D = MPPT(V,I)
% Perturb and observe on the boost duty cycle.
% A higher duty lowers the PV voltage, since Vpv = Vdc*(1-D).
Dmin = 0.45; Dmax = 0.8; D0 = 0.6375; dD = 0.003;
persistent Vold Pold Dold;
if isempty(Vold)
    Vold = V; Pold = V*I; Dold = D0;
end
P = V*I; dV = V - Vold; dP = P - Pold;
D = Dold;
if dP ~= 0
    if (dP > 0) == (dV > 0)
        D = Dold - dD;   % raise the voltage
    else
        D = Dold + dD;   % lower the voltage
    end
end
D = min(max(D, Dmin), Dmax);
Dold = D; Vold = V; Pold = P;
